simulink model "resonant_simu"  (R2019b)
settings: Solver=VariableStepAuto  StartTime=0.0  StopTime=simulation_time  RelTol=1e-3
values from neighbouring files (symbols this model uses):
  Gs = tf(0.5, [1 1])    [param2.m]    (also in params1.m = tf(b, [1 a]); params3.m = tf([b1 b0], [1 a1 a0]); resonant_params.m = tf(100, [1 10 0]); resonant_params2.m = tf([b1 b0], [1 a1 a0]))
  ResonantController = tf([c2 c1 c0], [1 0 w0^2])    [resonant_params.m]    (also in resonant_params2.m)
  Rm = 3    [resonant_params.m]    (also in resonant_params2.m)
  sampling_time = 0.001    [resonant_params.m]    (also in resonant_params2.m = 0.1)
  w0 = sqrt(2)    [resonant_params.m]    (also in resonant_params2.m)
settings Model: Creator=adityaaaap  LastModifiedBy=adityaaaap
settings OptimizationCC: DefaultParameterBehavior=Inlined  EnhancedBackFolding=on  PassReuseOutputArgsAs=Individual arguments  ZeroExternalMemoryAtStartup=off  ZeroInternalMemoryAtStartup=off  OptimizeBlockOrder=speed  DifferentSizesBufferReuse=on  OptimizationCustomize=off  EfficientTunableParamExpr=on
settings DebuggingCC: ParameterTunabilityLossMsg=error
settings SFSimCC: MATLABDynamicMemAlloc=off
settings RTWCC: SystemTargetFile=ert.tlc  GenCodeOnly=on  TemplateMakefile=ert_default_tmf  GenerateReport=on  IncludeHyperlinkInReport=on  LaunchReport=on  GenerateTraceInfo=on  GenerateTraceReport=on  GenerateTraceReportSl=on  GenerateTraceReportSf=on  GenerateTraceReportEml=on
settings CodeAppCC: ForceParamTrailComments=on  IgnoreCustomStorageClasses=off  OperatorAnnotations=on  SimulinkDataObjDesc=on  SFDataObjDesc=on  InsertBlockDesc=on
settings ERTTargetCC: TargetLangStandard=C99 (ISO)  GenerateSampleERTMain=on  InlinedParameterPlacement=NonHierarchical  ERTCustomFileTemplate=example_file_process.tlc

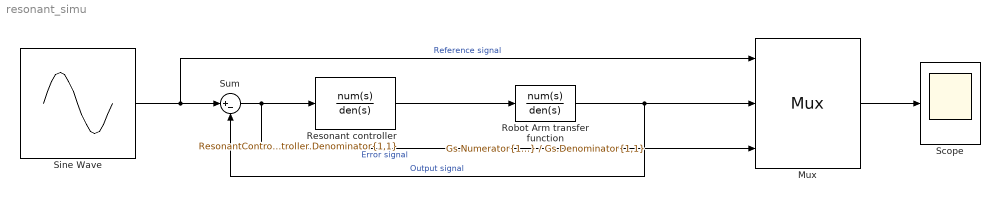
== system resonant_simu ==
  Mux : Mux  Inputs=3
      settings: DisplayOption=signals
  Resonant controller : TransferFcn  Numerator=ResonantController.Numerator{1,1}  Denominator=ResonantController.Denominator{1,1}
  Robot Arm transfer function : TransferFcn  Numerator=Gs.Numerator{1,1}  Denominator=Gs.Denominator{1,1}
  Scope : Scope
  Sine Wave : Sin  Amplitude=Rm  Frequency=w0  SampleTime=sampling_time
  Sum : Sum  Inputs=|+-
  wires:
  Sine Wave/1 -> Mux/1, Sum/1  "Reference signal"
  Sum/1 -> Mux/3, Resonant controller/1  "Error signal"
  Resonant controller/1 -> Robot Arm transfer function/1
  Mux/1 -> Scope/1
  Robot Arm transfer function/1 -> Mux/2, Sum/2  "Output signal"
